simulink model "NetraAI_DigitalTwin_V7_Working"  (Simulink 8.3)
settings: Solver=VariableStepDiscrete  StartTime=0.0  StopTime=28800  MaxStep=1  RelTol=1e-3
Description:
  | ANEYE / NetraAI Digital Twin V6. Primary and recapture acquisition traffic are merged using a SimEvents Path Combiner. Route-5 cases consume recapture preparation, a second fundus capture and a second AI pass. Recapture cases exit after the second AI pass; post-recapture clinical outcome is not inferred.
settings Model: Creator=kaustav  LastModifiedBy=kaustav
settings DataIOCC: SignalLoggingSaveFormat=Dataset
settings DebuggingCC: UnderspecifiedInitializationDetection=Simplified  StateNameClashWarn=none
settings GRTTargetCC: CombineOutputUpdateFcns=on  GRTInterface=off

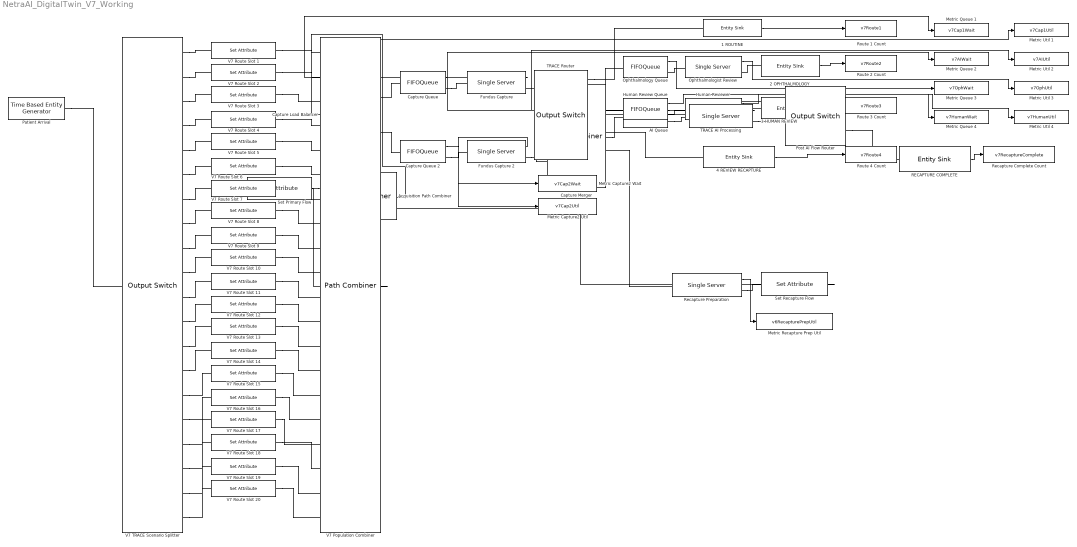
== system NetraAI_DigitalTwin_V7_Working ==
  1 ROUTINE : EntitySink  StatNumberArrived=on
  2 OPHTHALMOLOGY : EntitySink  StatNumberArrived=on
  3 HUMAN REVIEW : EntitySink  StatNumberArrived=on
  4 REVIEW RECAPTURE : EntitySink  StatNumberArrived=on
  AI Queue : FIFOQueue  Capacity=1000  StatAverageWait=on
      settings: OutputPortMap=o2
  Acquisition Path Combiner : PathCombiner  NumberInputPorts=2
  Capture Load Balancer : OutputSwitch  NumberOutputPorts=2  SwitchingCriterion=Round robin
  Capture Merger : PathCombiner  NumberInputPorts=2
  Capture Queue : FIFOQueue  Capacity=1000  StatAverageWait=on
      settings: OutputPortMap=o2
  Capture Queue 2 : FIFOQueue  Capacity=1000  StatAverageWait=on
      settings: OutputPortMap=o2
  Fundus Capture : SingleServer  ServiceTime=120  StatUtilization=on
      settings: OutputPortMap=o5
  Fundus Capture 2 : SingleServer  ServiceTime=120  StatUtilization=on
      settings: OutputPortMap=o5
  Human Review Queue : FIFOQueue  Capacity=1000  StatAverageWait=on
      settings: OutputPortMap=o2
  Human Reviewer : SingleServer  ServiceTime=45  StatUtilization=on
      settings: OutputPortMap=o5
  Metric Capture2 Util : ToWorkspace  VariableName=v7Cap2Util  SampleTime=-1
  Metric Capture2 Wait : ToWorkspace  VariableName=v7Cap2Wait  SampleTime=-1
  Metric Queue 1 : ToWorkspace  VariableName=v7Cap1Wait  SampleTime=-1
  Metric Queue 2 : ToWorkspace  VariableName=v7AIWait  SampleTime=-1
  Metric Queue 3 : ToWorkspace  VariableName=v7OphWait  SampleTime=-1
  Metric Queue 4 : ToWorkspace  VariableName=v7HumanWait  SampleTime=-1
  Metric Recapture Prep Util : ToWorkspace  VariableName=v6RecapturePrepUtil  SampleTime=-1
  Metric Util 1 : ToWorkspace  VariableName=v7Cap1Util  SampleTime=-1
  Metric Util 2 : ToWorkspace  VariableName=v7AIUtil  SampleTime=-1
  Metric Util 3 : ToWorkspace  VariableName=v7OphUtil  SampleTime=-1
  Metric Util 4 : ToWorkspace  VariableName=v7HumanUtil  SampleTime=-1
  Ophthalmologist Review : SingleServer  ServiceTime=30  StatUtilization=on
      settings: OutputPortMap=o5
  Ophthalmology Queue : FIFOQueue  Capacity=1000  StatAverageWait=on
      settings: OutputPortMap=o2
  Patient Arrival : TimeBasedEntityGenerator  Period=86.4
  Post AI Flow Router : OutputSwitch  NumberOutputPorts=2  SwitchingCriterion=From attribute  AttributeName=flowType
  RECAPTURE COMPLETE : EntitySink  StatNumberArrived=on
  Recapture Complete Count : ToWorkspace  VariableName=v7RecaptureComplete  SampleTime=-1
  Recapture Preparation : SingleServer  ServiceTime=20  StatUtilization=on
      settings: OutputPortMap=o5
  Route 1 Count : ToWorkspace  VariableName=v7Route1  SampleTime=-1
  Route 2 Count : ToWorkspace  VariableName=v7Route2  SampleTime=-1
  Route 3 Count : ToWorkspace  VariableName=v7Route3  SampleTime=-1
  Route 4 Count : ToWorkspace  VariableName=v7Route4  SampleTime=-1
  Set Primary Flow : SetAttribute  AttributeName=flowType  EvaluatedAttributeValue={ 1}
  Set Recapture Flow : SetAttribute  AttributeName=flowType  AttributeValue=2  EvaluatedAttributeValue={ 2}
  TRACE AI Processing : SingleServer  ServiceTime=8.67151  StatUtilization=on
      settings: OutputPortMap=o5
  TRACE Router : OutputSwitch  NumberOutputPorts=5  SwitchingCriterion=From attribute  AttributeName=routeCode
  V7 Population Combiner : PathCombiner  NumberInputPorts=20
  V7 Route Slot {1,7,13,19} (4 alike) : SetAttribute  AttributeName=routeCode  EvaluatedAttributeValue={ 1}
  V7 Route Slot 10 : SetAttribute  AttributeName=routeCode  AttributeValue=3  EvaluatedAttributeValue={ 3}
  V7 Route Slot 11 : SetAttribute  AttributeName=routeCode  AttributeValue=4  EvaluatedAttributeValue={ 4}
  V7 Route Slot {2,5,8,12,15,18} (6 alike) : SetAttribute  AttributeName=routeCode  AttributeValue=5  EvaluatedAttributeValue={ 5}
  V7 Route Slot {3,9,14,20} (4 alike) : SetAttribute  AttributeName=routeCode  AttributeValue=2  EvaluatedAttributeValue={ 2}
  V7 Route Slot 16 : SetAttribute  AttributeName=routeCode  AttributeValue=3  EvaluatedAttributeValue={ 3}
  V7 Route Slot 17 : SetAttribute  AttributeName=routeCode  AttributeValue=4  EvaluatedAttributeValue={ 4}
  V7 Route Slot 4 : SetAttribute  AttributeName=routeCode  AttributeValue=3  EvaluatedAttributeValue={ 3}
  V7 Route Slot 6 : SetAttribute  AttributeName=routeCode  AttributeValue=4  EvaluatedAttributeValue={ 4}
  V7 TRACE Scenario Splitter : OutputSwitch  NumberOutputPorts=20  SwitchingCriterion=Round robin
  wires:
  1 ROUTINE/1 -> Route 1 Count/1
  2 OPHTHALMOLOGY/1 -> Route 2 Count/1
  3 HUMAN REVIEW/1 -> Route 3 Count/1
  4 REVIEW RECAPTURE/1 -> Route 4 Count/1
  Capture Queue/1 -> Metric Queue 1/1
  AI Queue/1 -> Metric Queue 2/1
  Ophthalmology Queue/1 -> Metric Queue 3/1
  Human Review Queue/1 -> Metric Queue 4/1
  Fundus Capture/1 -> Metric Util 1/1
  TRACE AI Processing/1 -> Metric Util 2/1
  Ophthalmologist Review/1 -> Metric Util 3/1
  Human Reviewer/1 -> Metric Util 4/1
  Capture Queue 2/1 -> Metric Capture2 Wait/1
  Fundus Capture 2/1 -> Metric Capture2 Util/1
  RECAPTURE COMPLETE/1 -> Recapture Complete Count/1
  Recapture Preparation/1 -> Metric Recapture Prep Util/1
  connections:
  Ophthalmology Queue/RConn1 -- Ophthalmologist Review/LConn1
  Ophthalmologist Review/RConn1 -- 2 OPHTHALMOLOGY/LConn1
  Human Review Queue/RConn1 -- Human Reviewer/LConn1
  Human Reviewer/RConn1 -- 3 HUMAN REVIEW/LConn1
  AI Queue/RConn1 -- TRACE AI Processing/LConn1
  TRACE AI Processing/RConn1 -- Post AI Flow Router/LConn1
  Patient Arrival/RConn1 -- V7 TRACE Scenario Splitter/LConn1
  V7 TRACE Scenario Splitter/RConn1 -- V7 Route Slot 1/LConn1
  V7 Route Slot 1/RConn1 -- V7 Population Combiner/LConn1
  V7 TRACE Scenario Splitter/RConn2 -- V7 Route Slot 2/LConn1
  V7 Route Slot 2/RConn1 -- V7 Population Combiner/LConn2
  V7 TRACE Scenario Splitter/RConn3 -- V7 Route Slot 3/LConn1
  V7 Route Slot 3/RConn1 -- V7 Population Combiner/LConn3
  V7 TRACE Scenario Splitter/RConn4 -- V7 Route Slot 4/LConn1
  V7 Route Slot 4/RConn1 -- V7 Population Combiner/LConn4
  V7 TRACE Scenario Splitter/RConn5 -- V7 Route Slot 5/LConn1
  V7 Route Slot 5/RConn1 -- V7 Population Combiner/LConn5
  V7 TRACE Scenario Splitter/RConn6 -- V7 Route Slot 6/LConn1
  V7 Route Slot 6/RConn1 -- V7 Population Combiner/LConn6
  V7 TRACE Scenario Splitter/RConn7 -- V7 Route Slot 7/LConn1
  V7 Route Slot 7/RConn1 -- V7 Population Combiner/LConn7
  V7 TRACE Scenario Splitter/RConn8 -- V7 Route Slot 8/LConn1
  V7 Route Slot 8/RConn1 -- V7 Population Combiner/LConn8
  V7 TRACE Scenario Splitter/RConn9 -- V7 Route Slot 9/LConn1
  V7 Route Slot 9/RConn1 -- V7 Population Combiner/LConn9
  V7 TRACE Scenario Splitter/RConn10 -- V7 Route Slot 10/LConn1
  V7 Route Slot 10/RConn1 -- V7 Population Combiner/LConn10
  V7 TRACE Scenario Splitter/RConn11 -- V7 Route Slot 11/LConn1
  V7 Route Slot 11/RConn1 -- V7 Population Combiner/LConn11
  V7 TRACE Scenario Splitter/RConn12 -- V7 Route Slot 12/LConn1
  V7 Route Slot 12/RConn1 -- V7 Population Combiner/LConn12
  V7 TRACE Scenario Splitter/RConn13 -- V7 Route Slot 13/LConn1
  V7 Route Slot 13/RConn1 -- V7 Population Combiner/LConn13
  V7 TRACE Scenario Splitter/RConn14 -- V7 Route Slot 14/LConn1
  V7 Route Slot 14/RConn1 -- V7 Population Combiner/LConn14
  V7 TRACE Scenario Splitter/RConn15 -- V7 Route Slot 15/LConn1
  V7 Route Slot 15/RConn1 -- V7 Population Combiner/LConn15
  V7 TRACE Scenario Splitter/RConn16 -- V7 Route Slot 16/LConn1
  V7 Route Slot 16/RConn1 -- V7 Population Combiner/LConn16
  V7 TRACE Scenario Splitter/RConn17 -- V7 Route Slot 17/LConn1
  V7 Route Slot 17/RConn1 -- V7 Population Combiner/LConn17
  V7 TRACE Scenario Splitter/RConn18 -- V7 Route Slot 18/LConn1
  V7 Route Slot 18/RConn1 -- V7 Population Combiner/LConn18
  V7 TRACE Scenario Splitter/RConn19 -- V7 Route Slot 19/LConn1
  V7 Route Slot 19/RConn1 -- V7 Population Combiner/LConn19
  V7 TRACE Scenario Splitter/RConn20 -- V7 Route Slot 20/LConn1
  V7 Route Slot 20/RConn1 -- V7 Population Combiner/LConn20
  V7 Population Combiner/RConn1 -- Set Primary Flow/LConn1
  Acquisition Path Combiner/RConn1 -- Capture Load Balancer/LConn1
  Capture Load Balancer/RConn1 -- Capture Queue/LConn1
  Capture Queue/RConn1 -- Fundus Capture/LConn1
  Fundus Capture/RConn1 -- Capture Merger/LConn1
  Capture Load Balancer/RConn2 -- Capture Queue 2/LConn1
  Capture Queue 2/RConn1 -- Fundus Capture 2/LConn1
  Fundus Capture 2/RConn1 -- Capture Merger/LConn2
  Capture Merger/RConn1 -- AI Queue/LConn1
  Set Primary Flow/RConn1 -- Acquisition Path Combiner/LConn1
  Set Recapture Flow/RConn1 -- Acquisition Path Combiner/LConn2
  Post AI Flow Router/RConn1 -- TRACE Router/LConn1
  Post AI Flow Router/RConn2 -- RECAPTURE COMPLETE/LConn1
  TRACE Router/RConn1 -- 1 ROUTINE/LConn1
  TRACE Router/RConn2 -- Ophthalmology Queue/LConn1
  TRACE Router/RConn3 -- Human Review Queue/LConn1
  TRACE Router/RConn4 -- 4 REVIEW RECAPTURE/LConn1
  TRACE Router/RConn5 -- Recapture Preparation/LConn1
  Recapture Preparation/RConn1 -- Set Recapture Flow/LConn1
